simulink model "V605_tabularMotorModel"  (R2025a)
settings: Solver=VariableStepAuto  StartTime=0.0  StopTime=10.0  RelTol=1e-3
model workspace (MAT data in the model file):
  Sig = Simulink.Signal
  Sig.Dimensions = -1
  Sig.DimensionsMode = 'auto'
  Sig.Complexity = 'auto'
  Sig.SampleTime = -1
  Sig.SamplingMode = 'auto'
  Sig.DataType = 'auto'
settings Model: Creator=Tristan  LastModifiedBy=Ayush_S

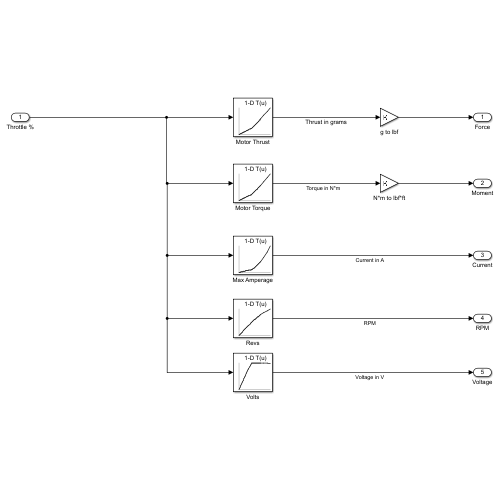
[thumbnail: Simulink's stored preview of the top-level diagram]
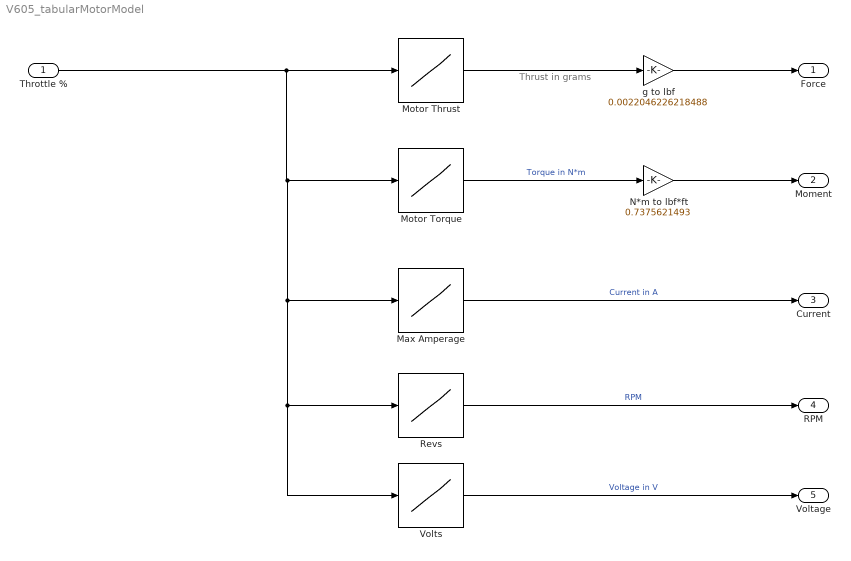
== system V605_tabularMotorModel ==
  note: Thrust in grams
  Throttle % : Inport
  Max Amperage : Lookup_n-D  NumberOfTableDimensions=1  BreakpointsForDimension1=[0;2;4;6;8;10;12;14;16;18;20;22;24;26;28;30;32;34;36;38;40;42;44;46;48;50;52;54;56;58;60;62;64;66;68;70;80;90;100]  Table=[0;0.35999999999999999;0.71999999999999997;1.0800000000000001;1.4399999999999999;1.8;2.1600000000000001;2.52;2.8799999999999999;3.2400000000000002;3.6099999999999999;3.9700000000000002;4.3300000000000001;4.6900000000000004;5.0499999999999998;5.4100000000000001;5.7699999999999996;6.1299999999999999;6.4900000000000002;6.8499999999999996;7.21;8.1999999999999993;9.0899999999999999;10.289999999999999;11.56;12.94;14.119999999999999;15.460000000000001;16.760000000000002;18;19.460000000000001;21.059999999999999;22.609999999999999;24.510000000000002;26.190000000000001;28.109999999999999;38.689999999999998;52.159999999999997;68.299999999999997]  InternalRulePriority=Speed  RndMeth=Simplest
  Motor Thrust : Lookup_n-D  NumberOfTableDimensions=1  BreakpointsForDimension1=[0;2;4;6;8;10;12;14;16;18;20;22;24;26;28;30;32;34;36;38;40;42;44;46;48;50;52;54;56;58;60;62;64;66;68;70;80;90;100]  Table=[0;145;290;435;580;725;869;1014;1159;1304;1449;1594;1739;1884;2029;2174;2318;2463;2608;2753;2898;3200;3464;3722;4059;4385;4663;4995;5266;5525;5788;6153;6455;6771;7049;7383;9108;10917;12761]  InternalRulePriority=Speed  RndMeth=Simplest
  Motor Torque : Lookup_n-D  NumberOfTableDimensions=1  BreakpointsForDimension1=[0;2;4;6;8;10;12;14;16;18;20;22;24;26;28;30;32;34;36;38;40;42;44;46;48;50;52;54;56;58;60;62;64;66;68;70;80;90;100]  Table=[0;0.040000000000000001;0.070000000000000007;0.11;0.14999999999999999;0.17999999999999999;0.22;0.26000000000000001;0.28999999999999998;0.33000000000000002;0.37;0.40000000000000002;0.44;0.46999999999999997;0.51000000000000001;0.55000000000000004;0.57999999999999996;0.62;0.66000000000000003;0.68999999999999995;0.72999999999999998;0.80000000000000004;0.85999999999999999;0.93000000000000005;1.02;1.0900000000000001;1.1599999999999999;1.24;1.3100000000000001;1.3600000000000001;1.4399999999999999;1.52;1.6000000000000001;1.6799999999999999;1.75;1.8400000000000001;2.2799999999999998;2.7999999999999998;3.2599999999999998]  InternalRulePriority=Speed  RndMeth=Simplest
  N*m to lbf*ft : Gain  Gain=0.7375621493
  Revs : Lookup_n-D  NumberOfTableDimensions=1  BreakpointsForDimension1=[0;2;4;6;8;10;12;14;16;18;20;22;24;26;28;30;32;34;36;38;40;42;44;46;48;50;52;54;56;58;60;62;64;66;68;70;80;90;100]  Table=[0;172;344;517;689;861;1033;1205;1378;1550;1722;1894;2066;2239;2411;2583;2755;2927;3100;3272;3444;3592;3762;3908;4063;4226;4352;4488;4618;4734;4859;4980;5107;5241;5363;5487;6025;6561;7036]  InternalRulePriority=Speed  RndMeth=Simplest
  Volts : Lookup_n-D  NumberOfTableDimensions=1  BreakpointsForDimension1=[0;2;4;6;8;10;12;14;16;18;20;22;24;26;28;30;32;34;36;38;40;42;44;46;48;50;52;54;56;58;60;62;64;66;68;70;80;90;100]  Table=[0;2.3999999999999999;4.79;7.1900000000000004;9.5800000000000001;11.98;14.369999999999999;16.77;19.16;21.559999999999999;23.949999999999999;26.350000000000001;28.739999999999998;31.140000000000001;33.530000000000001;35.93;38.32;40.719999999999999;43.109999999999999;45.509999999999998;47.899999999999999;47.880000000000003;47.859999999999999;47.829999999999998;47.799999999999997;47.770000000000003;47.75;47.719999999999999;47.700000000000003;47.670000000000002;47.630000000000003;47.600000000000001;47.579999999999998;47.530000000000001;47.490000000000002;47.450000000000003;47.229999999999997;46.950000000000003;46.600000000000001]  InternalRulePriority=Speed  RndMeth=Simplest
  g to lbf : Gain  Gain=0.0022046226218488
  Force : Outport
  Moment : Outport  Port=2
  Current : Outport  Port=3
  RPM : Outport  Port=4
  Voltage : Outport  Port=5
  wires:
  Motor Thrust/1 -> g to lbf/1
  Throttle %/1 -> Volts/1, Revs/1, Max Amperage/1, Motor Torque/1, Motor Thrust/1
  Motor Torque/1 -> N*m to lbf*ft/1  "Torque in N*m"
  Volts/1 -> Voltage/1  "Voltage in V"
  Revs/1 -> RPM/1  "RPM"
  Max Amperage/1 -> Current/1  "Current in A"
  g to lbf/1 -> Force/1
  N*m to lbf*ft/1 -> Moment/1
